simulink model "RWIP_nonlinear_model"  (R2025a)
settings: Solver=FixedStepAuto  StartTime=0.0  StopTime=10.0  FixedStep=1e-3  RelTol=1e-3
values from neighbouring files (symbols this model uses):
  dphi0 = 0    [config_model.m]
  dtheta0 = 0    [config_model.m]
  g = 9.81    [config_model.m]
  I_t = I_b + I_w + l_b^2 * m_b    (= 0.0241666666667)    [config_model.m]
  I_w = 1/2 * m_w * l_w^2    (= 0.0025)    [config_model.m]
  l_b = 0.2    [config_model.m]
  M = m_w + 1/2 * m_b    (= 0.75)    [config_model.m]
  phi0 = 0    [config_model.m]
  theta0 = pi/2    (= 1.57079632679)    [config_model.m]
settings Model: Creator=amoralesma  LastModifiedBy=amoralesma

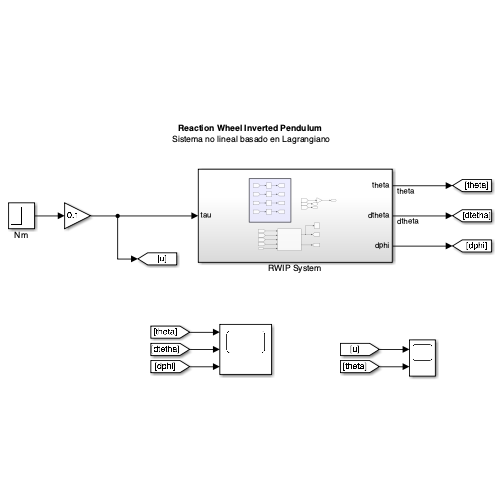
[thumbnail: Simulink's stored preview of the top-level diagram]
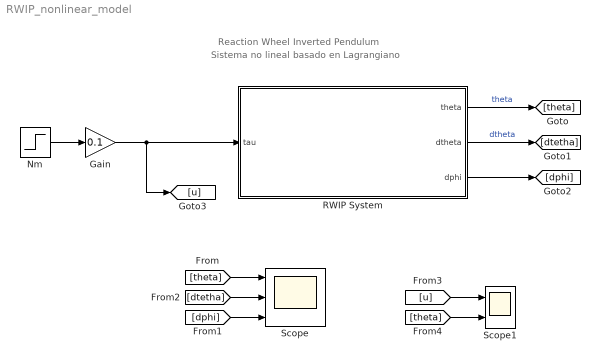
== system RWIP_nonlinear_model ==
  note: Reaction Wheel Inverted Pendulum
  note: Sistema no lineal basado en Lagrangiano
  Gain : Gain  Gain=0.1
  Nm : Step  Time=5  SampleTime=0
  RWIP System : Subsystem
  Scope : Scope  NumInputPorts=3
      settings: Title=Angular velocity (dtheta)  ActiveDisplayYMinimum=-14.715189797304525  ActiveDisplayYMaximum=14.715186388599832  YLabel=Angular velocity (rad/s)
  Scope1 : Scope  NumInputPorts=2
      settings: ActiveDisplayYMinimum=-0.012499999999999997  ActiveDisplayYMaximum=0.1125  DataLoggingVariableName=ScopeData2
  wires:
  Nm/1 -> Gain/1
  Gain/1 -> [u], RWIP System/1(tau)
  RWIP System/1(theta) -> [theta]  "theta"
  RWIP System/2(dtheta) -> [dtetha]  "dtheta"
  RWIP System/3(dphi) -> [dphi]
  [theta] -> Scope/1
  [dphi] -> Scope/3
  [dtetha] -> Scope/2
  [u] -> Scope1/1
  [theta] -> Scope1/2

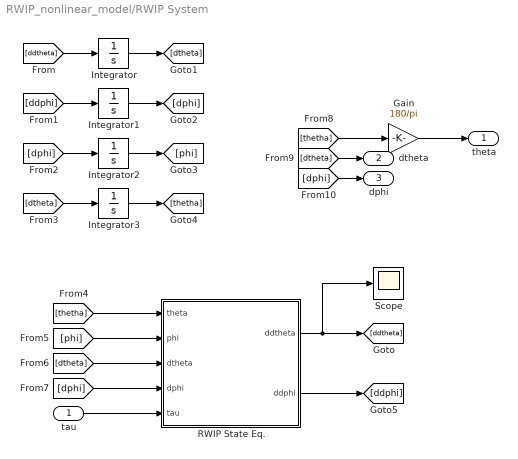
== system RWIP_nonlinear_model/RWIP System ==
  tau : Inport
  Gain : Gain  Gain=180/pi
  Integrator : Integrator  InitialCondition=dtheta0
  Integrator1 : Integrator  InitialCondition=dphi0
  Integrator2 : Integrator  InitialCondition=phi0
  Integrator3 : Integrator  InitialCondition=theta0
  RWIP State Eq. : MATLAB Function  TreatAsAtomicUnit=on
  Scope : Scope
      settings: ActiveDisplayYMinimum=-84.92475640283817  ActiveDisplayYMaximum=84.897622506298248
  theta : Outport
  dtheta : Outport  Port=2
  dphi : Outport  Port=3
  wires:
  [ddtheta] -> Integrator/1
  [dphi] -> Integrator2/1
  [dtheta] -> Integrator3/1
  Integrator2/1 -> [phi]
  Integrator1/1 -> [dphi]
  [ddphi] -> Integrator1/1
  Integrator/1 -> [dtheta]
  Integrator3/1 -> [thetha]
  [thetha] -> RWIP State Eq./1(theta)
  [phi] -> RWIP State Eq./2(phi)
  [dtheta] -> RWIP State Eq./3(dtheta)
  [dphi] -> RWIP State Eq./4(dphi)
  tau/1 -> RWIP State Eq./5(tau)
  RWIP State Eq./1(ddtheta) -> Scope/1, [ddtheta]
  RWIP State Eq./2(ddphi) -> [ddphi]
  [thetha] -> Gain/1
  [dtheta] -> dtheta/1
  [dphi] -> dphi/1
  Gain/1 -> theta/1

== matlab function RWIP_nonlinear_model/RWIP System/RWIP State Eq. ==
  data: theta input; ddtheta output; phi input; dtheta input; ddphi output; dphi input; tau input; l_b parameter; I_t parameter; M parameter; g parameter; I_w parameter
function [ddtheta, ddphi] = fcn(theta, phi, dtheta, dphi, tau, l_b, I_t, M, g, I_w)
  % Matriz de inercia
    Mmat = [I_t, I_w;
            I_w, I_w];

    % Término gravitacional
    G = [M*g*l_b*sin(theta);
          0];

    % Torque interno del reaction wheel
    B = [-1;
          1];

    % Visocidad 
    C = [ -dtheta * 0.001; 
        0]; 


    % Aceleraciones generalizadas
    qdd = Mmat \ (G + C + B*tau);

    ddtheta = qdd(1);
    ddphi   = qdd(2);
end
